simulink model "IC"  (Simulink 5.0)
settings: Solver=ode45  StartTime=0.0  StopTime=10.0  RelTol=1e-3
undefined symbols (not defined in the file or in its folder): T
settings Model: LastModifiedBy=dsplab

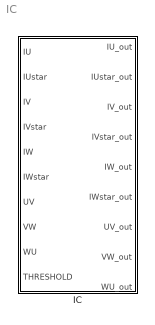
== system IC ==
  IC : Subsystem

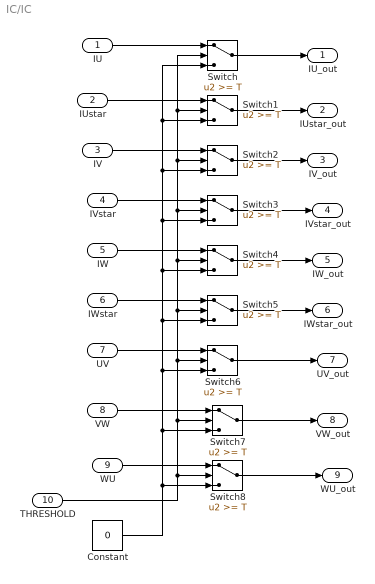
== system IC/IC ==
  IU : Inport
  IUstar : Inport  Port=2
  IV : Inport  Port=3
  IVstar : Inport  Port=4
  IW : Inport  Port=5
  IWstar : Inport  Port=6
  UV : Inport  Port=7
  VW : Inport  Port=8
  WU : Inport  Port=9
  THRESHOLD : Inport  Port=10
  Constant : Constant  Value=0
  Switch{,1..8} (9 alike) : Switch  Threshold=T  SaturateOnIntegerOverflow=on
  IU_out : Outport
  IUstar_out : Outport  Port=2
  IV_out : Outport  Port=3
  IVstar_out : Outport  Port=4
  IW_out : Outport  Port=5
  IWstar_out : Outport  Port=6
  UV_out : Outport  Port=7
  VW_out : Outport  Port=8
  WU_out : Outport  Port=9
  wires:
  IU/1 -> Switch/1
  IUstar/1 -> Switch1/1
  IV/1 -> Switch2/1
  IVstar/1 -> Switch3/1
  IW/1 -> Switch4/1
  IWstar/1 -> Switch5/1
  UV/1 -> Switch6/1
  VW/1 -> Switch7/1
  WU/1 -> Switch8/1
  Constant/1 -> Switch8/3, Switch7/3, Switch6/3, Switch5/3, Switch4/3, Switch3/3, Switch2/3, Switch1/3, Switch/3
  Switch/1 -> IU_out/1
  Switch1/1 -> IUstar_out/1
  Switch2/1 -> IV_out/1
  Switch3/1 -> IVstar_out/1
  Switch4/1 -> IW_out/1
  Switch5/1 -> IWstar_out/1
  Switch6/1 -> UV_out/1
  Switch7/1 -> VW_out/1
  Switch8/1 -> WU_out/1
  THRESHOLD/1 -> Switch/2, Switch1/2, Switch2/2, Switch3/2, Switch4/2, Switch5/2, Switch6/2, Switch7/2, Switch8/2
